simulink model "convergenzak"  (R2022a)
settings: Solver=VariableStepAuto  StartTime=0.0  StopTime=10  RelTol=1e-3
values from neighbouring files (symbols this model uses):
  T_gps = 14*T    [gain_p.m]    (also in init.m = 0.25)
settings Model: Creator=morel  LastModifiedBy=Leo
settings ModelReferenceCC: EnableRefExpFcnMdlSchedulingChecks=off
settings RTWCC: Description=Generic Real-Time Target

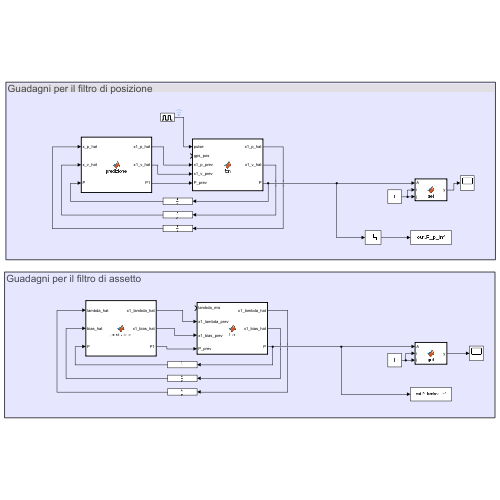
[thumbnail: Simulink's stored preview of the top-level diagram]
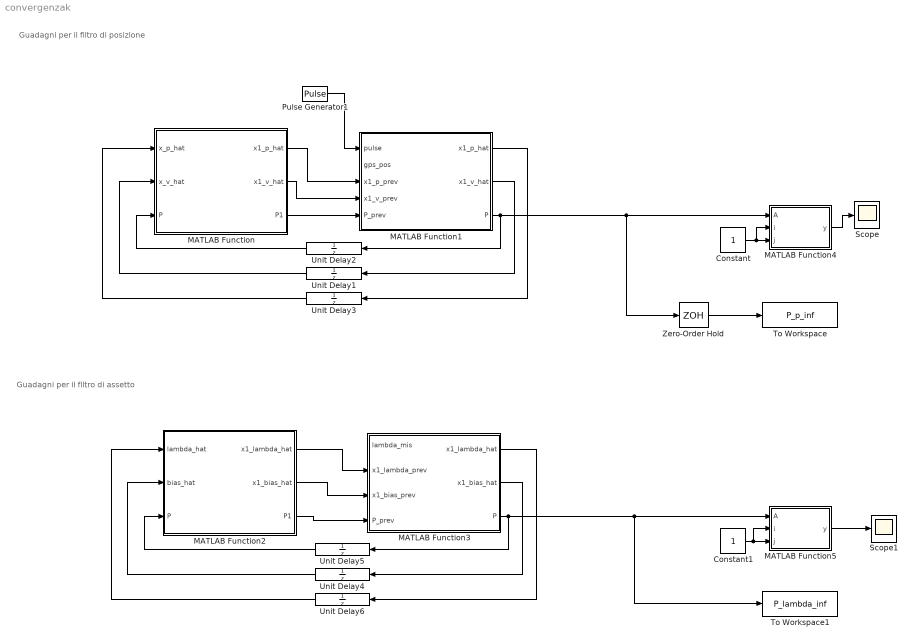
== system convergenzak ==
  note: Guadagni per il filtro di assetto
  note: Guadagni per il filtro di posizione
  Constant : Constant
  Constant1 : Constant
  MATLAB Function : MATLAB Function  TreatAsAtomicUnit=on
  MATLAB Function1 : MATLAB Function  TreatAsAtomicUnit=on
  MATLAB Function2 : MATLAB Function  TreatAsAtomicUnit=on
  MATLAB Function3 : MATLAB Function  TreatAsAtomicUnit=on
  MATLAB Function4 : MATLAB Function  TreatAsAtomicUnit=on
  MATLAB Function5 : MATLAB Function  TreatAsAtomicUnit=on
  Pulse Generator1 : DiscretePulseGenerator  PulseType=Time based  Period=1/4  PulseWidth=10
  Scope : Scope
  Scope1 : Scope
  To Workspace : ToWorkspace  VariableName=P_p_inf  SampleTime=-1
  To Workspace1 : ToWorkspace  VariableName=P_lambda_inf  SampleTime=-1
  Unit Delay{1,3..4,6} (4 alike) : UnitDelay  InitialCondition=zeros(3,1)  SampleTime=-1  HasFrameUpgradeWarning=on
  Unit Delay2 : UnitDelay  InitialCondition=10*eye(6)  SampleTime=-1  HasFrameUpgradeWarning=on
  Unit Delay5 : UnitDelay  InitialCondition=0.02*eye(6)  SampleTime=-1  HasFrameUpgradeWarning=on
  Zero-Order Hold : ZeroOrderHold  SampleTime=T_gps
  wires:
  Pulse Generator1/1 -> MATLAB Function1/1(pulse)
  MATLAB Function/1(x1_p_hat) -> MATLAB Function1/3(x1_p_prev)
  MATLAB Function/2(x1_v_hat) -> MATLAB Function1/4(x1_v_prev)
  MATLAB Function/3(P1) -> MATLAB Function1/5(P_prev)
  MATLAB Function1/2(x1_v_hat) -> Unit Delay1/1
  MATLAB Function1/1(x1_p_hat) -> Unit Delay3/1
  Unit Delay2/1 -> MATLAB Function/3(P)
  Unit Delay1/1 -> MATLAB Function/2(x_v_hat)
  Unit Delay3/1 -> MATLAB Function/1(x_p_hat)
  MATLAB Function1/3(P) -> Zero-Order Hold/1, MATLAB Function4/1(A), Unit Delay2/1
  MATLAB Function3/3(P) -> MATLAB Function5/1(A), To Workspace1/1, Unit Delay5/1
  MATLAB Function3/1(x1_lambda_hat) -> Unit Delay6/1
  Unit Delay6/1 -> MATLAB Function2/1(lambda_hat)
  Unit Delay4/1 -> MATLAB Function2/2(bias_hat)
  Unit Delay5/1 -> MATLAB Function2/3(P)
  MATLAB Function2/1(x1_lambda_hat) -> MATLAB Function3/2(x1_lambda_prev)
  MATLAB Function2/3(P1) -> MATLAB Function3/4(P_prev)
  MATLAB Function3/2(x1_bias_hat) -> Unit Delay4/1
  MATLAB Function2/2(x1_bias_hat) -> MATLAB Function3/3(x1_bias_prev)
  MATLAB Function4/1(y) -> Scope/1
  MATLAB Function5/1(y) -> Scope1/1
  Constant/1 -> MATLAB Function4/2(i), MATLAB Function4/3(j)
  Constant1/1 -> MATLAB Function5/2(i), MATLAB Function5/3(j)
  Zero-Order Hold/1 -> To Workspace/1

== matlab function convergenzak/MATLAB Function1 ==
  settings: updateMethod=DISCRETE  sampleTime=T
  data: pulse input; gps_pos input; x1_p_prev input; x1_p_hat output; x1_v_prev input; P_prev input; x1_v_hat output; P output
function [x1_p_hat, x1_v_hat,P] = fcn(pulse,gps_pos,x1_p_prev, x1_v_prev,P_prev)

%% Gestione delle misure dei sensori e inizializzazione
    % pulse = 1 -> arriva una nuova misura del sensore
    % pulse = 0 -> non c'è nessuna nuova misura
  
    % Stato predetto in ingresso
    xi_prev = [x1_p_prev ; x1_v_prev];

    if pulse == 1  
        % Jacobiani del modello di misura rispetto allo stato e ai rumori
        H = [eye(3), zeros(3,3)];
        M = eye(3);
        % Digonale matrice di covarianza dei rumori sulle misure
        R = eye(3); 
        % innovazione
        e = gps_pos-x1_p_prev;

        %% Applico la correzione
            S = H*P_prev*H' + M*R*M';         % Matrice covarianza innovazione     
            L = P_prev*H'/S;                  % Guadagno correzione

            % Stato corretto ->  X_k|k
                xi_hat = xi_prev + L*e;  
            % Matrice di covarianza associata alla stima -> P_k|k 
                P = (eye(6) - L*H)*P_prev*(eye(6) - L*H)' + L*M*R*M'*L';  

           
    else  
           % Stato corretto ->  X_k|k
                xi_hat = xi_prev;  
            % Matrice di covarianza associata alla stima -> P_k|k 
                P = P_prev;  
    end

    %% Output blocco di correzione 
    x1_p_hat = xi_hat(1:3,:);
    x1_v_hat = xi_hat(4:end,:);
end

== matlab function convergenzak/MATLAB Function ==
  settings: updateMethod=DISCRETE  sampleTime=T
  data: x_p_hat input; x1_p_hat output; x_v_hat input; x1_v_hat output; P1 output; P input; T parameter
function [x1_p_hat, x1_v_hat,P1] = predizione(x_p_hat,x_v_hat,P,T)

F = [   eye(3),     T*eye(3);
      zeros(3,3),    eye(3)  ];

G = [   eye(3),   -T^2/2*eye(3);
      zeros(3,3),    T*eye(3)  ];

% Disturbi posizione 
sigma_p = 5*10^-2*eye(3);
sigma_a = 10 *eye(3);

sigma = [sigma_p zeros(3,3); zeros(3,3) sigma_a];

wpk = zeros(3,1);
wvk = zeros(3,1);


x1 = F*[x_p_hat ; x_v_hat] + G *[ wpk; wvk ];

x1_p_hat = x1(1:3,:);
x1_v_hat = x1(4:end,:);


P1 = F*P*F' + G*sigma*G';

== matlab function convergenzak/MATLAB Function2 ==
  settings: updateMethod=DISCRETE  sampleTime=T
  data: lambda_hat input; x1_lambda_hat output; bias_hat input; x1_bias_hat output; P1 output; P input; T parameter
function [x1_lambda_hat, x1_bias_hat,P1] = predizione(lambda_hat,bias_hat,P,T)

F = [   eye(3),     -T*eye(3);
      zeros(3,3),    eye(3)  ];

G = [ -T*eye(3),   zeros(3,3);
      zeros(3,3),    T*eye(3)  ];

% Rumore
    
% Disturbi posizione 
sigma_w = 3*eye(3);
sigma_b = 1e-10 *eye(3);

sigma = [sigma_w zeros(3,3); zeros(3,3) sigma_b];

wpk = zeros(3,1);
wvk = zeros(3,1);


x1 = F*[lambda_hat ; bias_hat] + G *[ wpk; wvk ];

x1_lambda_hat = x1(1:3,:);
x1_bias_hat = x1(4:end,:);


P1 = F*P*F' + G*sigma*G';

== matlab function convergenzak/MATLAB Function3 ==
  settings: updateMethod=DISCRETE  sampleTime=T
  data: lambda_mis input; x1_lambda_prev input; x1_lambda_hat output; x1_bias_prev input; P_prev input; x1_bias_hat output; P output
function [x1_lambda_hat, x1_bias_hat,P] = fcn(lambda_mis,x1_lambda_prev, x1_bias_prev,P_prev)

%% Gestione delle misure dei sensori e inizializzazione
    % pulse = 1 -> arriva una nuova misura del sensore
    % pulse = 0 -> non c'è nessuna nuova misura
  
    % Stato predetto in ingresso
    xi_prev = [x1_lambda_prev ; x1_bias_prev];

        % Jacobiani del modello di misura rispetto allo stato e ai rumori
        H = [eye(3), zeros(3,3)];
        M = eye(3);
        % Digonale matrice di covarianza dei rumori sulle misure
        R = 0.8e-2*eye(3); 
        % innovazione
        e = lambda_mis-x1_lambda_prev;

        %% Applico la correzione
            S = H*P_prev*H' + M*R*M';         % Matrice covarianza innovazione     
            L = P_prev*H'/S;                  % Guadagno correzione

            % Stato corretto ->  X_k|k
                xi_hat = xi_prev + L*e;  
            % Matrice di covarianza associata alla stima -> P_k|k 
                P = (eye(6) - L*H)*P_prev*(eye(6) - L*H)' + L*M*R*M'*L';  

    %% Output blocco di correzione 
    x1_lambda_hat = xi_hat(1:3,:);
    x1_bias_hat = xi_hat(4:end,:);
end

== matlab function convergenzak/MATLAB Function4 ==
  data: A input; y output; i input; j input
function y = get(A,i,j)
y = A(i,j);

== matlab function convergenzak/MATLAB Function5 ==
  data: A input; y output; i input; j input
function y = get(A,i,j)
y = A(i,j);
